simulink model "example_CollectorUnglazed"  (R2018b)
settings: Solver=ode45  StartTime=0.0  StopTime=24*3600  RelTol=1e-5  AbsTol=1e-5  EnableMultiTasking=on
undefined symbols (not defined in the file): path_carnot
libraries: carnot x5
settings Model: Creator=drhf  LastModifiedBy=drhf
settings SolverCC: AutoScaleAbsTol=off
settings DataIOCC: LimitDataPoints=on  SaveFormat=Array
settings OptimizationCC: ExpressionDepthLimit=2147483647  LifeSpan=inf
settings DebuggingCC: UnderspecifiedInitializationDetection=Classic  MergeDetectMultiDrivingBlocksExec=none  SolverPrmCheckMsg=warning  StateNameClashWarn=warning  SFUnexpectedBacktrackingDiag=warning  SFNoUnconditionalDefaultTransitionDiag=warning  SFExecutionAtInitializationDiag=none
settings HardwareCC: ProdBitPerPointer=32  ProdBitPerSizeT=32  ProdBitPerPtrDiffT=32  ProdLargestAtomicFloat=None  ProdIntDivRoundTo=Undefined  ProdEndianess=Unspecified  ProdWordSize=32  ProdHWDeviceType=32-bit Generic
settings ModelReferenceCC: PropagateSignalLabelsOutOfModel=off
settings SFSimCC: SimUseLocalCustomCode=off
settings RTWCC: RTWUseLocalCustomCode=off
settings CodeAppCC: StateflowObjectComments=on
settings GRTTargetCC: TargetLangStandard=C89/C90 (ANSI)  GeneratePreprocessorConditionals=Disable all  CombineOutputUpdateFcns=off  GRTInterface=on
settings ConfigComp: CovMetricSettings=dw  CovHtmlReporting=on  CovSaveCumulativeToWorkspaceVar=on  CovSaveSingleToWorkspaceVar=on  CovExternalEMLEnable=off

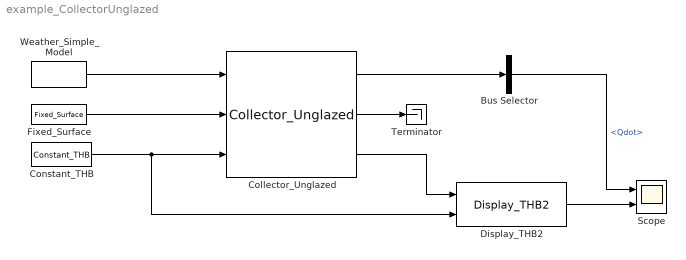
== system example_CollectorUnglazed ==
  Bus Selector : BusSelector  OutputSignals=Qdot
  Collector_Unglazed : carnot/Source/Solar_Thermal/Collector_Unglazed  tini=20  Ncollector=1  PathName=fullfile(path_carnot('libsl'), 'Source', 'Solar_Thermal', 'Collector_Unglazed', 'parameter_set')  FileName='DefaultCollectorUnglazed.mat'  userPath=off  userParam=off  acol=2.5  len=2.3  nodes=5  fta=0.75  eps=0.9  u0l=4  u0c=10  u0g=4  u1l=3  u1c=3  u1g=1.5  u1e=0.01  hi=100  capa=7000  capf=2000  SensorTimeConstant=10  dplin=10  dpqua=10
  Constant_THB : carnot/Source/Simple/Constant_THB  t=40  mdot=100/3600  p=1e5  mID=No Pressure Drop  fluid=Water  mix=0  mix2=0  mix3=0  dia=0.02  hgt=0
  Display_THB2 : carnot/Outputs/Display_THB2  t=on  m=off  p=off  id=off  mix=off  d=off
  Fixed_Surface : carnot/Weather/Fixed_Surface  colangle=30  colazi=0  colrot=0
  Scope : Scope  NumInputPorts=2
  Terminator : Terminator
  Weather_Simple_Model : carnot/Weather/Weather_Simple_Model  lat=60  Ibn=900  Idg=100  tamb=5  deltaTsky=-6  rh=50  precip="10e-3/24/3600           % 10 mm in 24 h"  cloud=0.125  p=1013e2  vw=1  wdir=270
  wires:
  Weather_Simple_Model/1 -> Collector_Unglazed/1
  Fixed_Surface/1 -> Collector_Unglazed/2
  Constant_THB/1 -> Collector_Unglazed/3, Display_THB2/2
  Collector_Unglazed/3 -> Display_THB2/1
  Display_THB2/1 -> Scope/2
  Collector_Unglazed/1 -> Bus Selector/1
  Bus Selector/1 -> Scope/1  "<Qdot>"
  Collector_Unglazed/2 -> Terminator/1
